simulink model "writer"  (R2020a)
settings: Solver=FixedStepDiscrete  StartTime=0.0  StopTime=0.6  FixedStep=0.1  RelTol=1e-3  EnableMultiTasking=on
settings Model: Creator=bzhan  LastModifiedBy=bzhan
settings SolverCC: AutoInsertRateTranBlk=on
settings DataIOCC: LimitDataPoints=on
settings OptimizationCC: LifeSpan=inf
settings DebuggingCC: AllowSymbolicDim=off  SFUnexpectedBacktrackingDiag=warning  SFNoUnconditionalDefaultTransitionDiag=warning  SFExecutionAtInitializationDiag=none  ArithmeticOperatorsInVariantConditions=warning
settings SFSimCC: SimUseLocalCustomCode=off  CustomCodeUndefinedFunction=UseInterfaceOnly
settings RTWCC: RTWUseLocalCustomCode=off
settings CodeAppCC: StateflowObjectComments=on
settings GRTTargetCC: TargetLangStandard=C89/C90 (ANSI)
settings ConfigComp: CovMetricSettings=dw  CovHtmlReporting=on  CovSaveCumulativeToWorkspaceVar=on  CovSaveSingleToWorkspaceVar=on  CovShowResultsExplorer=off  CovExternalEMLEnable=off  CovSFcnEnable=off

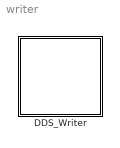
== system writer ==
  DDS_Writer : Stateflow chart  TreatAsAtomicUnit=on

== stateflow chart writer/DDS_Writer ==
  state add
    du: g()
  (default) -> add : {i=1;first_SN=1;last_SN=0;}
  add -> add : [i<=5]
      | {WHC(i)=cachechanges(i);first_SN=1;
      | last_SN=i;i = i + 1;f()}
  data: i local int8; WHC local =[0,0,0,0,0]; cachechanges local =[100,200,300,400,500]; first_SN local int8; last_SN local int8
  function g:
    | function g()
    |   fprintf("%.0f,%.0f,%.0f,%.0f,%.0f\n", WHC(1), WHC(2), WHC(3), WHC(4), WHC(5));
  function f:
    | function f()
    |   fprintf("%d,%d\n", first_SN, last_SN);
